simulink model "UnitTest_BusEval"  (R2020a)
settings: Solver=ode1  StartTime=0.0  StopTime=12  FixedStep=Ts_BigModel.Ts_base  MaxStep=Ts  RelTol=1e-3
undefined symbols (not defined in the file or in its folder): mode, pitch, roll, throttle, tilt_anglein, yaw
settings Model: Creator=sl  LastModifiedBy=Administrator
settings DataIOCC: SaveOutput=off  SaveTime=off
settings OptimizationCC: DefaultParameterBehavior=Inlined  EnhancedBackFolding=on  PassReuseOutputArgsAs=Individual arguments  ZeroExternalMemoryAtStartup=off  ZeroInternalMemoryAtStartup=off  OptimizeBlockOrder=speed  DifferentSizesBufferReuse=on  OptimizationCustomize=off  EfficientTunableParamExpr=on
settings DebuggingCC: InheritedTsInSrcMsg=none  ParameterPrecisionLossMsg=none  ParameterTunabilityLossMsg=error  UnconnectedInputMsg=none  UnconnectedOutputMsg=none  UnconnectedLineMsg=none
settings HardwareCC: ProdBitPerPointer=32  ProdBitPerSizeT=32  ProdBitPerPtrDiffT=32  ProdLargestAtomicInteger=Long  ProdLargestAtomicFloat=Double  ProdWordSize=32  ProdHWDeviceType=ARM Compatible->ARM Cortex
settings ModelReferenceCC: ParallelModelReferenceMATLABWorkerInit=Copy Base Workspace  ModelReferenceNumInstancesAllowed=Single
settings SFSimCC: MATLABDynamicMemAlloc=off
settings RTWCC: SystemTargetFile=ert.tlc  GenCodeOnly=on  PackageGeneratedCodeAndArtifacts=on  TemplateMakefile=ert_default_tmf  GenerateReport=on  IncludeHyperlinkInReport=on  LaunchReport=on  GenerateTraceInfo=on  GenerateTraceReport=on  GenerateTraceReportSl=on  GenerateTraceReportSf=on  GenerateTraceReportEml=on
settings CodeAppCC: ForceParamTrailComments=on  IgnoreCustomStorageClasses=off  MaxIdLength=48  OperatorAnnotations=on  SimulinkDataObjDesc=on  SFDataObjDesc=on  MATLABFcnDesc=on  InsertBlockDesc=on  MATLABSourceComments=on
settings ERTTargetCC: TargetLangStandard=C99 (ISO)  GenerateSampleERTMain=on  LogVarNameModifier=none  SupportVariableSizeSignals=on  InlinedParameterPlacement=NonHierarchical  ERTCustomFileTemplate=example_file_process.tlc  ERTFilePackagingFormat=Compact

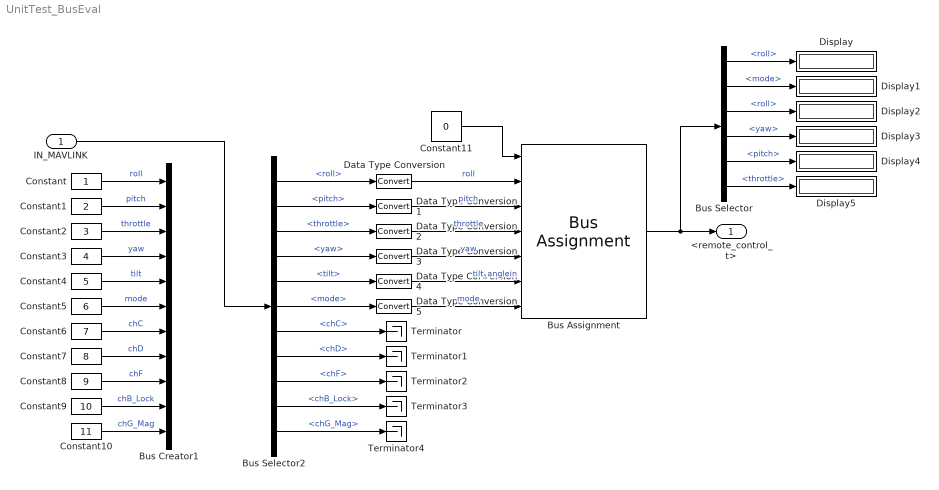
== system UnitTest_BusEval ==
  IN_MAVLINK : Inport  OutDataTypeStr=Bus: BUS_MAVLINK_TO_FIRM  BusOutputAsStruct=on
  Bus Assignment : BusAssignment  AssignedSignals=roll,pitch,throttle,yaw,tilt_anglein,mode
  Bus Creator1 : BusCreator  Inputs=11
  Bus Selector : BusSelector  OutputSignals=roll,mode,roll,yaw,pitch,throttle
  Bus Selector2 : BusSelector  OutputSignals=remote_control_t.roll,remote_control_t.pitch,remote_control_t.throttle,remote_control_t.yaw,remote_control_t.tilt,remote_control_t.mode,remote_control_t.chC,remote_control_t.chD,remote_control_t.chF,remote_control_t.chB_Lock,remote_control_t.chG_Mag
  Constant : Constant
  Constant1 : Constant  Value=2
  Constant10 : Constant  Value=11
  Constant11 : Constant  Value=0  OutDataTypeStr=Bus: BUS_CTRL_remote_ct_st
  Constant2 : Constant  Value=3
  Constant3 : Constant  Value=4
  Constant4 : Constant  Value=5
  Constant5 : Constant  Value=6
  Constant6 : Constant  Value=7
  Constant7 : Constant  Value=8
  Constant8 : Constant  Value=9
  Constant9 : Constant  Value=10
  Data Type Conversion{,1..5} (6 alike) : DataTypeConversion
  Display{,1..5} (6 alike) : Display
  Terminator{,1..4} (5 alike) : Terminator
  <remote_control_t> : Outport  OutDataTypeStr=Bus: BUS_CTRL_remote_ct_st  BusOutputAsStruct=on
  wires:
  Bus Assignment/1 -> Bus Selector/1, <remote_control_t>/1
  Bus Selector2/7 -> Terminator/1  "<chC>"
  Bus Selector2/11 -> Terminator4/1  "<chG_Mag>"
  Bus Selector2/8 -> Terminator1/1  "<chD>"
  Bus Selector2/9 -> Terminator2/1  "<chF>"
  Bus Selector2/10 -> Terminator3/1  "<chB_Lock>"
  Constant/1 -> Bus Creator1/1  "roll"
  Constant1/1 -> Bus Creator1/2  "pitch"
  Constant2/1 -> Bus Creator1/3  "throttle"
  Constant3/1 -> Bus Creator1/4  "yaw"
  Constant4/1 -> Bus Creator1/5  "tilt"
  Constant5/1 -> Bus Creator1/6  "mode"
  Constant6/1 -> Bus Creator1/7  "chC"
  Constant7/1 -> Bus Creator1/8  "chD"
  Constant8/1 -> Bus Creator1/9  "chF"
  Constant9/1 -> Bus Creator1/10  "chB_Lock"
  Constant10/1 -> Bus Creator1/11  "chG_Mag"
  Bus Selector/1 -> Display/1  "<roll>"
  Bus Selector/2 -> Display1/1  "<mode>"
  Bus Selector/3 -> Display2/1  "<roll>"
  Bus Selector/4 -> Display3/1  "<yaw>"
  Bus Selector/5 -> Display4/1  "<pitch>"
  Bus Selector/6 -> Display5/1  "<throttle>"
  IN_MAVLINK/1 -> Bus Selector2/1
  Bus Selector2/1 -> Data Type Conversion/1  "<roll>"
  Bus Selector2/2 -> Data Type Conversion1/1  "<pitch>"
  Bus Selector2/3 -> Data Type Conversion2/1  "<throttle>"
  Bus Selector2/4 -> Data Type Conversion3/1  "<yaw>"
  Bus Selector2/5 -> Data Type Conversion4/1  "<tilt>"
  Bus Selector2/6 -> Data Type Conversion5/1  "<mode>"
  Constant11/1 -> Bus Assignment/1
  Data Type Conversion2/1 -> Bus Assignment/4  "throttle"
  Data Type Conversion4/1 -> Bus Assignment/6  "tilt_anglein"
  Data Type Conversion1/1 -> Bus Assignment/3  "pitch"
  Data Type Conversion3/1 -> Bus Assignment/5  "yaw"
  Data Type Conversion/1 -> Bus Assignment/2  "roll"
  Data Type Conversion5/1 -> Bus Assignment/7  "mode"
